simulink model "untitled4"  (Simulink 7.7)
settings: Solver=ode45  StartTime=0.0  StopTime=10.0  RelTol=1e-3
settings Model: Creator=güler  LastModifiedBy=güler

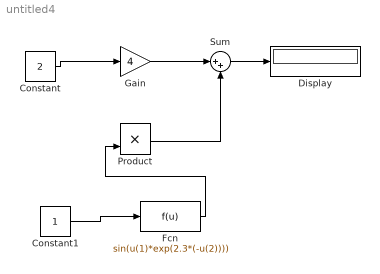
== system untitled4 ==
  Constant : Constant  Value=2
  Constant1 : Constant
  Display : Display
  Fcn : Fcn  Expr=sin(u(1)*exp(2.3*(-u(2))))
  Gain : Gain  Gain=4
  Product : Product  RndMeth=Zero
  Sum : Sum  Inputs=|++
  wires:
  Gain/1 -> Sum/1
  Product/1 -> Sum/2
  Sum/1 -> Display/1
  Constant/1 -> Gain/1
  ? -> ?
  Fcn/1 -> Product/2
  Constant1/1 -> Fcn/1
